simulink model "DCMotor1"  (Simulink 7.5)
settings: Solver=ode45  StartTime=0.0  StopTime=1  RelTol=1e-3
libraries: powerlib x3
settings Model: Creator=lm  LastModifiedBy=lm

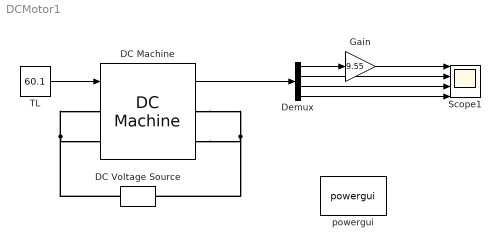
== system DCMotor1 ==
  DC Machine : powerlib/Machines/DC Machine  DialogController=POWERSYS.PowerSysDialog  SystemSampleTime=-1  PresetModel=No  MechanicalLoad=Torque TL  FieldType=Wound  ShowDetailedParameters=on  RLa="[ 0.087  0.0032]"  RLf="[ 181.5  0]"  Laf=0.56  MachineConstant=Torque constant (N.m/A)  Ke=1.8  Kt=1.8  J=0.76  Bm=0  Tf=0  w0=0  Ifinit=1  TsPowergui=0  TsBlock=-1
      settings: AttributesFormatString=\n
  DC Voltage Source : powerlib/Electrical Sources/DC Voltage Source  DialogController=POWERSYS.PowerSysDialog  SystemSampleTime=-1  Amplitude=220  Measurements=None
  Demux : Demux
  Gain : Gain  Gain=9.55  ParameterDataType=fixdt(1, 16)  ParameterScaling=2^0  OutDataType=fixdt(1, 16)  OutScaling=2^0
  Scope1 : Scope  NumInputPorts=4
      settings: YMin=-5~50~-5~-5  YMax=5~300~5~5
  TL : Constant  Value=60.1  OutDataType=fixdt(1, 16)  OutScaling=2^0
  powergui : powerlib/powergui  Priority=1  SystemSampleTime=-1  SimulationMode=Continuous  SampleTime=50e-6  frequency=60  SPID=off  DisableSnubberDevices=off  DisableRonSwitches=off  DisableVfSwitches=off  SwTol=0  Interpol=off  frequencyindice=0  echomessages=off  HookPort=off  DisplayEquations=off  FunctionMessages=off  EnableUseOfTLC=off  x0status=blocks  RestoreLinks=warning  ResistiveCurrentMeasurement=off  Ylog=off  Xlog=on  ShowGrid=off  save=off  variable=ZData  ZoomFFT=off  StartTime=0.0  cycles=1  DisplayStyle=1  FreqAxis=off  MaxFrequency=1000  frequencyindicesteady=1  display=off  methode=off
  wires:
  DC Machine/1 -> Demux/1
  TL/1 -> DC Machine/1
  Demux/1 -> Gain/1
  Gain/1 -> Scope1/1
  Demux/2 -> Scope1/2
  Demux/3 -> Scope1/3
  Demux/4 -> Scope1/4
  connections:
  DC Voltage Source/RConn1 -- DC Machine/LConn1 -- DC Machine/LConn2
  DC Machine/RConn1 -- DC Voltage Source/LConn1 -- DC Machine/RConn2
